simulink model "model"  (R2018a)
settings: Solver=VariableStepAuto  StartTime=0.0  StopTime=3  FixedStep=0.0001  RelTol=1e-3
PostLoadFcn:
  | cd(fileparts(which(bdroot)))
InitFcn:
  | initdata
values from neighbouring files (symbols this model uses):
  mu = xlsread('mu.xlsx','A1:A21')    [initdata.m]
  slip = xlsread('slip.xlsx','A1:A21')    [initdata.m]
settings Model: ModifiedByFormat=Mars  ModifiedHistory=Modified by YiXiuKeJi; Taobao is : https://shop197632247.taobao.com  Creator=一休科技  LastModifiedBy=Mars
settings SolverCC: ZeroCrossAlgorithm=Adaptive
settings DebuggingCC: MaxConsecutiveZCsMsg=none
settings CodeAppCC: StateflowObjectComments=on

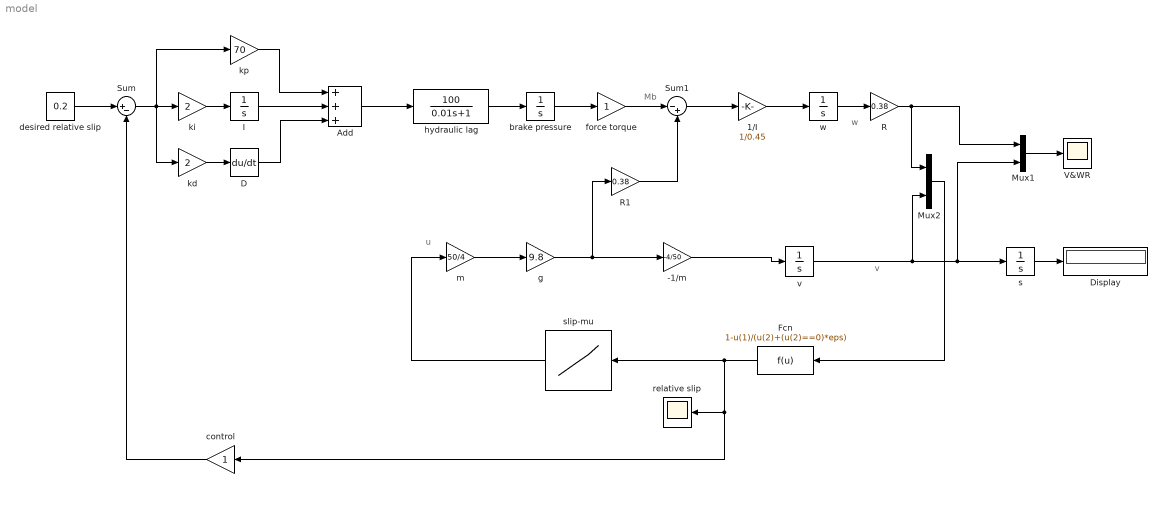
== system model ==
  note: Mb
  note: v
  note: w
  note: u
  -1/m : Gain  Gain=-4/50
  1/I : Gain  Gain=1/0.45
  Add : Sum  Inputs=+++
  D : Derivative
  Display : Display
  Fcn : Fcn  Expr=1-u(1)/(u(2)+(u(2)==0)*eps)
  I : Integrator
  Mux1 : Mux  Inputs=2
  Mux2 : Mux  Inputs=2
  R : Gain  Gain=0.38
  R1 : Gain  Gain=0.38
  Sum : Sum  Inputs=|+-
  Sum1 : Sum  Inputs=|-+
  V&WR : Scope
  brake pressure : Integrator  LimitOutput=on  UpperSaturationLimit=1500  LowerSaturationLimit=0
  control : Gain
  desired relative slip : Constant  Value=0.2
  force torque : Gain
  g : Gain  Gain=9.8
  hydraulic lag : TransferFcn  Numerator=[100]  Denominator=[0.01 1]
  kd : Gain  Gain=2
  ki : Gain  Gain=2
  kp : Gain  Gain=70
  m : Gain  Gain=50/4
  relative slip : Scope
  s : Integrator
  slip-mu : Lookup_n-D  NumberOfTableDimensions=1  BreakpointsForDimension1=slip  Table=mu  InternalRulePriority=Speed  RndMeth=Simplest  InputSameDT=on
  v : Integrator  InitialCondition=60/3.6  LimitOutput=on  UpperSaturationLimit=1000  LowerSaturationLimit=0
  w : Integrator  InitialCondition=60/3.6/0.38  LimitOutput=on  UpperSaturationLimit=1000  LowerSaturationLimit=0
  wires:
  Sum/1 -> ki/1, kd/1, kp/1
  desired relative slip/1 -> Sum/1
  ki/1 -> I/1
  1/I/1 -> w/1
  w/1 -> R/1
  v/1 -> Mux2/2, Mux1/2, s/1
  R/1 -> Mux2/1, Mux1/1
  kp/1 -> Add/1
  hydraulic lag/1 -> brake pressure/1
  Mux2/1 -> Fcn/1
  s/1 -> Display/1
  D/1 -> Add/3
  slip-mu/1 -> m/1
  Fcn/1 -> control/1, relative slip/1, slip-mu/1
  Mux1/1 -> V&WR/1
  kd/1 -> D/1
  R1/1 -> Sum1/2
  Add/1 -> hydraulic lag/1
  control/1 -> Sum/2
  Sum1/1 -> 1/I/1
  brake pressure/1 -> force torque/1
  force torque/1 -> Sum1/1
  m/1 -> g/1
  I/1 -> Add/2
  g/1 -> R1/1, -1/m/1
  -1/m/1 -> v/1
